simulink model "Impedance_Control"  (R2022a)
settings: Solver=VariableStepAuto  StartTime=0.0  StopTime=10.0  RelTol=1e-3
settings Model: Creator=dariu  LastModifiedBy=dariu
settings ModelReferenceCC: EnableRefExpFcnMdlSchedulingChecks=off
settings RTWCC: Description=Generic Real-Time Target

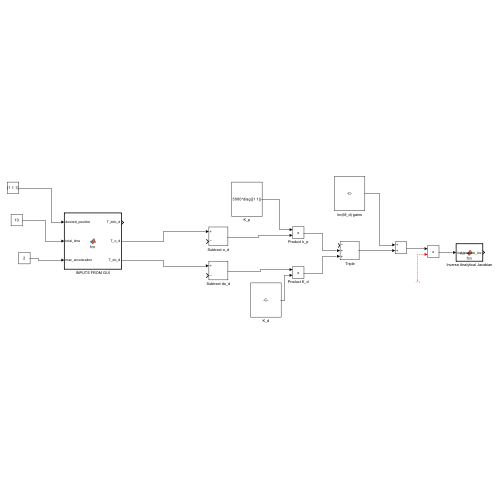
[thumbnail: Simulink's stored preview of the top-level diagram]
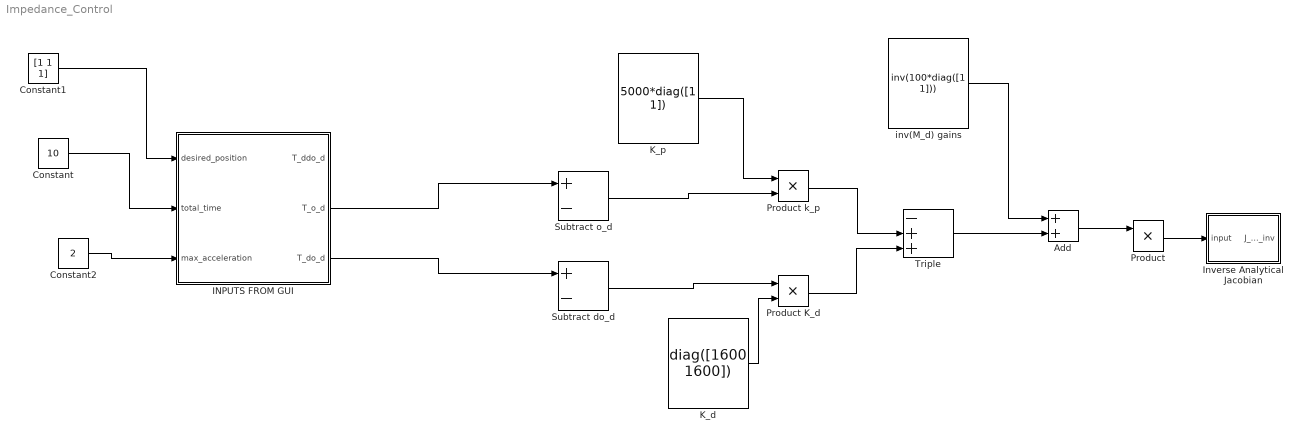
== system Impedance_Control ==
  " Triple" : Sum  Inputs=-++
  Add : Sum
  Constant : Constant  Value=10
  Constant1 : Constant  Value=[1 1 1]
  Constant2 : Constant  Value=2
  INPUTS FROM GUI : MATLAB Function  TreatAsAtomicUnit=on
  Inverse Analytical Jacobian : MATLAB Function  TreatAsAtomicUnit=on
  K_d : Constant  Value=diag([1600 1600])
  K_p : Constant  Value=5000*diag([1 1])
  Product : Product
  Product K_d : Product
  Product k_p : Product
  Subtract do_d : Sum  Inputs=+-
  Subtract o_d : Sum  Inputs=+-
  inv(M_d) gains : Constant  Value=inv(100*diag([1 1]))
  wires:
  Subtract do_d/1 -> Product K_d/1
  K_d/1 -> Product K_d/2
  Subtract o_d/1 -> Product k_p/2
  K_p/1 -> Product k_p/1
  Product K_d/1 -> " Triple"/3
  Product k_p/1 -> " Triple"/2
  " Triple"/1 -> Add/2
  inv(M_d) gains/1 -> Add/1
  Add/1 -> Product/1
  ? -> Product/2
  Product/1 -> Inverse Analytical Jacobian/1(input)
  INPUTS FROM GUI/2(T_o_d) -> Subtract o_d/1
  INPUTS FROM GUI/3(T_do_d) -> Subtract do_d/1
  Constant/1 -> INPUTS FROM GUI/2(total_time)
  Constant1/1 -> INPUTS FROM GUI/1(desired_position)
  Constant2/1 -> INPUTS FROM GUI/3(max_acceleration)

== matlab function Impedance_Control/INPUTS FROM GUI ==
  data: T_ddo_d output; T_o_d output; T_do_d output; desired_position input; total_time input; max_acceleration input
function [T_ddo_d, T_o_d, T_do_d] = fcn(desired_position, total_time, max_acceleration)
    % disp(thetas{1})
    % %T0H = f_kinematics(control_thetas, control_alphas, control_as, control_ds);
    T0H = f_kinematics(thetas, alphas, a, d);
    % INITIAL END EFFECTOR POSITION
    p_i = T0H(1:3, 4);
    
    % DESIRED END EFFECTOR POSITION
    p_f = desired_position;
    
    % Time settings
    T = total_time;
    T_a = T/5;
    a_max = max_acceleration;
    v_max = a_max * T_a;

    t = linspace(0, T, 1000);
    o_d = zeros(size(t));
    do_d = zeros(size(t));
    ddo_d = zeros(size(t));

    for i = 1:length(t)
        if t(i) < T_a
            % Acceleration phase
            o_d(i) = p_i + 0.5 * a_max * t(i)^2;
            do_d(i) = a_max * t(i);
            ddo_d(i) = a_max;
        elseif t(i) < (T - T_a)
            % Constant velocity phase
            o_d(i) = p_i + v_max * (t(i) - T_a) + 0.5 * a_max * T_a^2;
            do_d(i) = v_max;
            ddo_d(i) = 0;
        else
            % Deceleration phase
            o_d(i) = p_f - 0.5 * a_max * (T - t(i))^2;
            do_d(i) = a_max * (T - t(i));
            ddo_d(i) = -a_max;
        end
    end
    T_o_d = [t', o_d'];
    T_do_d = [t', do_d'];
    T_ddo_d = [t', ddo_d'];

end

== matlab function Impedance_Control/Inverse Analytical Jacobian ==
  data: input input; J_pseudo_inv output
function J_pseudo_inv = fcn(input)
    J_a = analytical_Ja(thetas, alphas, as, ds);
    J_pseudo = pinv(J_a);
    J_pseudo_inv = subs(J_pseudo, thetas, control_thetas);
    J_pseudo_inv = subs(J_pseudo_inv, alphas, control_alphas);
    J_pseudo_inv = subs(J_pseudo_inv, as, control_as);
    J_pseudo_inv = subs(J_pseudo_inv, ds, control_ds);

end
